simulink model "Three_Level_Inverter"  (R2020b)
settings: Solver=VariableStepAuto  StartTime=0.0  StopTime=0.02  FixedStep=1e-9  RelTol=1e-3
model workspace (MAT data in the model file):
  Tri_wave_dt = 2.5e-05
  Ts = 2e-06
libraries: ee_lib x55, nesl_utility x29, fl_lib x28, simulink x2
(part 2 of 2)

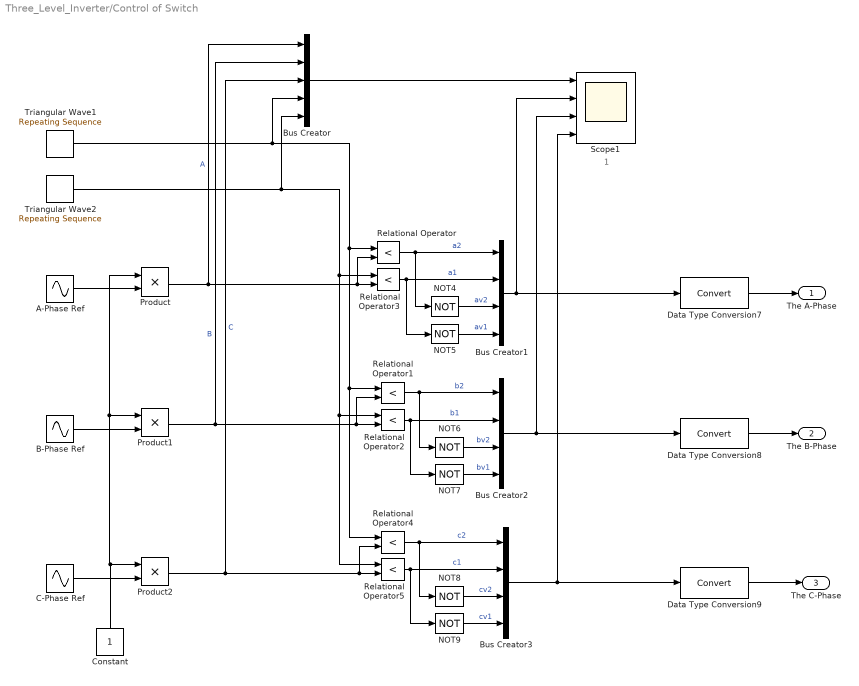
== system Three_Level_Inverter/Control of Switch ==
  note: 1
  A-Phase Ref : Sin  Frequency=2*pi*50  SampleTime=0
  B-Phase Ref : Sin  Frequency=2*pi*50  Phase=2*pi/3  SampleTime=0
  Bus Creator : BusCreator  Inputs=5
  Bus Creator1 : BusCreator  Inputs=4
  Bus Creator2 : BusCreator  Inputs=4
  Bus Creator3 : BusCreator  Inputs=4
  C-Phase Ref : Sin  Frequency=2*pi*50  Phase=-2*pi/3  SampleTime=0
  Constant : Constant
  Data Type Conversion7 : DataTypeConversion
  Data Type Conversion8 : DataTypeConversion
  Data Type Conversion9 : DataTypeConversion
  NOT{4..9} (6 alike) : Logic  Operator=NOT  IconShape=distinctive  AllPortsSameDT=off  OutDataTypeStr=boolean
  Product : Product
  Product1 : Product
  Product2 : Product
  Relational Operator{,1..5} (6 alike) : RelationalOperator  Operator=<  OutDataTypeStr=boolean  RndMeth=Simplest
  Scope1 : Scope  NumInputPorts=4
  Triangular Wave1 : simulink/Sources/Repeating Sequence  rep_seq_t=[0 Tri_wave_dt 2*Tri_wave_dt]  rep_seq_y=[0 1 0]
  Triangular Wave2 : simulink/Sources/Repeating Sequence  rep_seq_t=[0 Tri_wave_dt 2*Tri_wave_dt]  rep_seq_y=[0 -1 0]
  The A-Phase : Outport
  The B-Phase : Outport  Port=2
  The C-Phase : Outport  Port=3
  wires:
  Bus Creator/1 -> Scope1/1
  A-Phase Ref/1 -> Product/2
  Constant/1 -> Product/1, Product1/1, Product2/1
  B-Phase Ref/1 -> Product1/2
  C-Phase Ref/1 -> Product2/2
  Product1/1 -> Bus Creator/2, Relational Operator1/2, Relational Operator2/2  "B"
  Relational Operator/1 -> NOT4/1, Bus Creator1/1  "a2"
  Product/1 -> Bus Creator/1, Relational Operator/2, Relational Operator3/2  "A"
  Bus Creator2/1 -> Scope1/3, Data Type Conversion8/1
  Bus Creator1/1 -> Scope1/2, Data Type Conversion7/1
  Data Type Conversion9/1 -> The C-Phase/1
  Data Type Conversion8/1 -> The B-Phase/1
  Data Type Conversion7/1 -> The A-Phase/1
  Relational Operator3/1 -> NOT5/1, Bus Creator1/2  "a1"
  NOT6/1 -> Bus Creator2/3  "bv2"
  Bus Creator3/1 -> Scope1/4, Data Type Conversion9/1
  NOT4/1 -> Bus Creator1/3  "av2"
  NOT5/1 -> Bus Creator1/4  "av1"
  Relational Operator5/1 -> Bus Creator3/2, NOT9/1  "c1"
  Triangular Wave1/1 -> Bus Creator/4, Relational Operator1/1, Relational Operator4/1, Relational Operator/1
  Product2/1 -> Bus Creator/3, Relational Operator4/2, Relational Operator5/2  "C"
  Relational Operator4/1 -> Bus Creator3/1, NOT8/1  "c2"
  NOT8/1 -> Bus Creator3/3  "cv2"
  NOT9/1 -> Bus Creator3/4  "cv1"
  NOT7/1 -> Bus Creator2/4  "bv1"
  Relational Operator2/1 -> Bus Creator2/2, NOT7/1  "b1"
  Relational Operator1/1 -> Bus Creator2/1, NOT6/1  "b2"
  Triangular Wave2/1 -> Bus Creator/5, Relational Operator2/1, Relational Operator5/1, Relational Operator3/1
